simulink library "CSWLibrary"  (R2021a)
settings: Solver=VariableStepAuto  StartTime=0.0  StopTime=10.0  RelTol=1e-3
settings Model: Creator=Martin  LastModifiedBy=Martin

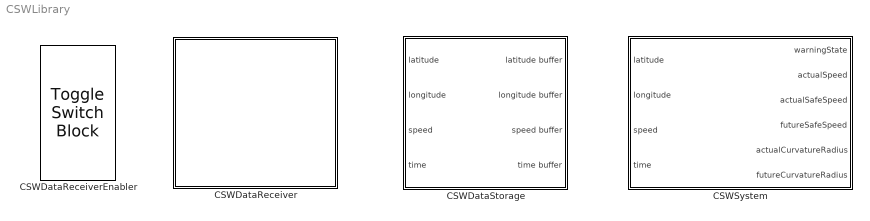
== system CSWLibrary ==
  CSWDataReceiver : MATLAB Function  TreatAsAtomicUnit=on  mask{inputPort=1, predictionTime=5, maximumLateralAcceleration=5.9, safeLimit=60, lowerRadius=20, upperRadius=600, isRunning=0, visualizeTrajectory=on, logReceivedData=on, receivedDataFile=output.xlsx, saveResults=on, simulationResultsFile=results.xlsx}
      mask prompts: inputPort "Serial port - COM"; predictionTime "Prediction time (s)"; maximumLateralAcceleration "Maximum lateral acceleration (m/s^2)"; safeLimit "Safe limit (0 -100%) of original Maximum lateral acceleration value"; lowerRadius "Lower limit (m)"; upperRadius "Upper limit (m)"; isRunning "Running"; visualizeTrajectory "Visualize trajectory - Future trajectory can be viewed by enabling checkbox."; logReceivedData "Log received data"; receivedDataFile "Received data file name (.xlsx)"; saveResults "Save simulation results"; simulationResultsFile "Results file name (.xlsx)"
      mask help:
      | CSWData receiver block of Curve Speed Warning System Toolbox processes received (online) GPS NMEA-0183 data from serial COM port. Data is used to simulate Curve Speed Warning system with options to visualize simulation, save received data and save simulation result data. Based on the input data, the system decides whether or not to give warning signal to driver. System is successfully initialized after getting 3 records containing correct input data.
      |
      | CSWData receiver block stops after CSWDataReceiver enabler block is set to Off value.
      |
      | CSWData receiver block expects online data.
  CSWDataReceiverEnabler : ToggleSwitchBlock
      settings: Values={{'Off', 'On'}, [0 1]}
  CSWDataStorage : Subsystem
      mask help:
      | CSWData storage block of Curve Speed Warning System Toolbox serves as storage for (offline) input data (latitude: double, longitude: double, speed: double, time: double) loaded from file, which are given as input data for CSWSystem block. Maximum capacity for each component of input data are 3 records.
      |
      | CSWData storage block is used to store offline data loaded from file.
  CSWSystem : MATLAB Function  TreatAsAtomicUnit=on  mask{predictionTime=5, maximumLateralAcceleration=5.9, safeLimit=60, lowerRadius=20, upperRadius=600, visualizeTrajectory=on, saveResults=on, simulationResultsFile=results.xlsx}
      mask prompts: predictionTime "Prediction time (s)"; maximumLateralAcceleration "Maximum lateral acceleration (m/s^2)"; safeLimit "Safe limit (0 -100%) of original Maximum lateral acceleration value"; lowerRadius "Lower limit (m)"; upperRadius "Upper limit (m)"; visualizeTrajectory "Visualize trajectory - Future trajectory can be viewed by enabling checkbox."; saveResults "Save simulation results"; simulationResultsFile "Results file name (.xlsx)"
      mask help:
      | System block of Curve Speed Warning System Toolbox processed input (offline) data (latitude: double, longitude: double, speed: double, time: double) from CSWData storage block to simulate Curve Speed Warning system. Data is used to simulate Curve Speed Warning system with options to visualize simulation and save simulation result data. Based on the input data, the system decides whether or not to give warning signal to driver. System is successfully initialized after getting 3 records containing correct input data.
      |
      | CSWSystem block expects offline data loaded from From Spreadsheet block with parameter Output after last data point set to Ground value.

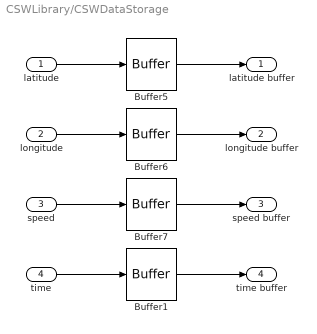
== system CSWLibrary/CSWDataStorage ==
  latitude : Inport
  longitude : Inport  Port=2
  speed : Inport  Port=3
  time : Inport  Port=4
  Buffer{1,5..7} (4 alike) : Buffer  N=3  V=2  ic=-199  OutputFrames=off
  latitude buffer : Outport
  longitude buffer : Outport  Port=2
  speed buffer : Outport  Port=3
  time buffer : Outport  Port=4
  wires:
  speed/1 -> Buffer7/1
  Buffer5/1 -> latitude buffer/1
  longitude/1 -> Buffer6/1
  Buffer7/1 -> speed buffer/1
  Buffer6/1 -> longitude buffer/1
  latitude/1 -> Buffer5/1
  time/1 -> Buffer1/1
  Buffer1/1 -> time buffer/1

== matlab function CSWLibrary/CSWSystem ==
  data: latitude input; longitude input; warningState output; actualSpeed output; actualSafeSpeed output; speed input; futureSafeSpeed output; actualCurvatureRadius output; futureCurvatureRadius output; time input
%% main function which represents Curve Speed Warning System uses loaded GPS data from file to compute simulation results which containts warning state, recommended speed etc.

function [warningState, actualSpeed, actualSafeSpeed, futureSafeSpeed, actualCurvatureRadius, futureCurvatureRadius] = CSWSystem(latitude,longitude,speed,time)
    coder.extrinsic('plot','legend','serialport','readline','nmeaParser','getfield','set_param','ceil','str2double',...
        'get_param','gcb','datetime');
    
    persistent predictionTime;  
    predictionTime = double(0);
    predictionTime = ceil(str2double(get_param(gcb,'predictionTime')));
    persistent maximumLateralAcceleration;
    maximumLateralAcceleration = double(0);
    maximumLateralAcceleration = str2double(get_param(gcb,'maximumLateralAcceleration'));
    persistent safeLimit;
    safeLimit = double(0);
    safeLimit = str2double(get_param(gcb,'safeLimit'));
    persistent lowerRadius;
    lowerRadius = double(0);
    lowerRadius = str2double(get_param(gcb,'lowerRadius'));
    persistent upperRadius;
    upperRadius = double(0);
    upperRadius = str2double(get_param(gcb,'upperRadius'));
    persistent visualizeTrajectory;
    visualizeTrajectory = str2bool(get_param(gcb,'visualizeTrajectory'));
    persistent saveResults;
    saveResults = str2bool(get_param(gcb,'saveResults'));
    
    % check if input data are valid
    validation(predictionTime, maximumLateralAcceleration, safeLimit, lowerRadius, upperRadius);
    
    % check if simulation results will be written to file
    persistent simulationResultsFile;  
    if(saveResults)
        simulationResultsFile = get_param(gcb,'simulationResultsFile');
        if(~endsWith(simulationResultsFile,'.xlsx'))
            error('Invalid simulation results file name format. Use .xlsx instead')
        end
    else
        simulationResultsFile = '-1';
    end

    persistent index;
    index = 3;
    
    data = [latitude(:) longitude(:) speed(:) time(:)];
    deltaTime12 = double(0);
    deltaTime23 = double(0);
    
    if ismember(-199, data)
        warningState = 0;
        actualSafeSpeed = -1;
        futureSafeSpeed = -1;
        actualCurvatureRadius = -1;
        futureCurvatureRadius = -1;
        actualSpeed = -1;
        return;
    end

    if (ismember(0, latitude(:)) && ismember(0, longitude(:)) && ismember(0, speed(:)) && ismember(0, time(:)))
        error('Input data contains an invalid zero value/s')
    end

    % convert coordinates to Cartesian coordinate system and center coordinates along Y axis
    data = centerDataArray(data);

    allData = [data(index - 2,1) data(index - 2,2) data(index - 2,3); 
        data(index - 1,1) data(index - 1,2) data(index - 1,3); 
        data(index,1) data(index,2) data(index,3)
        ];
    predictedData = [data(index,1) data(index,2) data(index,3)];

    tempData = [
        data(length(data(:,1))-2,1) data(length(data(:,1))-2,2) data(length(data(:,1))-2,3) data(length(data(:,1))-2,4);
        data(length(data(:,1))-1,1) data(length(data(:,1))-1,2) data(length(data(:,1))-1,3) data(length(data(:,1))-1,4); 
        data(length(data(:,1)),1) data(length(data(:,1)),2) data(length(data(:,1)),3) data(length(data(:,1)),4)
        ];
    
    % decode time values
    time1 = datetime(time(1),'ConvertFrom','posixtime', 'Format', 'yyyy-MM-dd HH:mm:ss');
    time2 = datetime(time(2),'ConvertFrom','posixtime', 'Format', 'yyyy-MM-dd HH:mm:ss');
    time3 = datetime(time(3),'ConvertFrom','posixtime', 'Format', 'yyyy-MM-dd HH:mm:ss');

    % differences between recording times
    deltaTime12 = seconds(diff(datetime([time1;time2])));
    deltaTime23 = seconds(diff(datetime([time2;time3])));
    
    % check validation of time differences (it's expected, that records will be received with same time frequency)
    if (deltaTime12 ~= deltaTime23)
        if(visualizeTrajectory)
            plot(0,0);
            title('invalid records, retrying...');
            set(gca, 'Color',[1 1 0]);
        end
        warningState = 0;
        actualSafeSpeed = -1;
        futureSafeSpeed = -1;
        actualCurvatureRadius = -1;
        futureCurvatureRadius = -1;
        actualSpeed = -1;
        return;
    end
    
    timeRate = deltaTime23;

    if (timeRate > 0)
        steps = 0;
        steps = ceil(predictionTime / timeRate);
        % prediction loop in which are future coordinates predicted
        for time = 1:steps
            [predictedX, predictedY] = predictCoordinates(tempData, 3, timeRate);  

            tempData = [tempData(2,1) tempData(2,2) tempData(2,3) tempData(2,4);
                tempData(3,1) tempData(3,2) tempData(3,3) tempData(3,4);
                predictedX predictedY getNextSpeed(tempData, 3) 0;
                ];

            allData = [allData; [tempData(3,1) tempData(3,2) tempData(3,3)]];
            predictedData = [predictedData; [tempData(3,1) tempData(3,2) tempData(3,3)]];
        end

        % compute radius and speed of actual and predicted data
        allData = computeCurvatureRadiusAndSpeed(allData,maximumLateralAcceleration*((100-safeLimit)/100));

        N = size(allData,1);
        allData = [allData,zeros(N,1)];

        % decide if warning should be invoked
        allData = checkCurvatureRadiusAndSpeed(allData, lowerRadius, upperRadius);
        
        % write results to file
        if(~isequal(simulationResultsFile,'-1'))
            writeResults(simulationResultsFile, allData, data(3,4));
        end

        actualSpeed = allData(3,3);
        actualSafeSpeed = allData(3,6);
        futureSafeSpeed = allData(4,6);
        actualCurvatureRadius = allData(3,5);
        futureCurvatureRadius = allData(4,5);

        if ismember(1, allData(:,7))
            warningState = 1;
        else
            warningState = 0;
        end
        
        % trajectory visualization containing referenced and predicted data
        if(visualizeTrajectory)
            plotOutput(allData, predictedData, timeRate);
        end
    else
        warningState = 0;
        actualSafeSpeed = -1;
        futureSafeSpeed = -1;
        actualCurvatureRadius = -1;
        futureCurvatureRadius = -1;
        actualSpeed = -1;
        return;
    end
end


%% convert string to boolean

function [output]=str2bool(string)
   if strcmp(string,'off')
     output = false;
   else
     output = true;
   end
end


%% input values validation

function validation(predictionTime, maximumLateralAcceleration, safeLimit, lowerRadius, upperRadius)
    if(predictionTime <= 0 || predictionTime > 30)
        error('Invalid value of prediction time. Valid value is from range 0(excluding) - 30')
    end
    
    if(maximumLateralAcceleration < 0)
        error('Negative value of maximum lateral acceleration is not supported')
    end
    
    if(safeLimit > 100 || safeLimit < 0)
        error('Invalid value of safe limit, set value in range 0 to 100')
    end
    
    if(lowerRadius < 0 || upperRadius < 0)
        error('Negative value of curvature radius limit is not supported')
    end

    if(lowerRadius > upperRadius)
        error('Lower limit of curvature radius must be smaller than upper limit')
    end
end


%% plot output prediction trajectory with / without warning

function plotOutput(allData, predictedData, timeRate)
    coder.extrinsic('plot','legend');
    
    % find maximum value among X,Y data points to specify size of plot figure
    xMin = min(allData(:,1)) - 5;
    xMax = max(allData(:,1)) + 5;
    
    x1 = abs(xMin);
    x2 = abs(xMax);
    
    xResult = x1;
    if(x1 < x2)
        xResult = x2;
    end
    
    yMin = min(allData(:,2)) - 5;
    yMax = max(allData(:,2)) + 5;
    
    y1 =  abs(yMin);
    y2 =  abs(yMax);
    
    yResult = y1;
    if(y1 < y2)
        yResult = y2;
    end
    
    result = 5;
    tempResult = yResult;
    if (yResult < xResult)
        tempResult = xResult;
    end
    if (result < tempResult)
        result = tempResult;
    end
    
    % plot output
    plot(allData(:,1), allData(:,2), 'b-o', 'DisplayName','referenced coordinates')
    xlim([-result result])
    ylim([yMin result])
    hold on
    plot(predictedData(:,1), predictedData(:,2), 'g-o', 'DisplayName','predicted coordinates')
    plot(predictedData(1,1), predictedData(1,2), 'k-o', 'DisplayName','actual position')
    
    % set frequency in which are points plotted in figure
    title(sprintf('point frequency is %.1f second/s',timeRate));
    
    % show figure legend
    legend('referenced coordinates','predicted coordinates','actual position')
    
    % set background color depending on warning state (warning - red background / no warning - white background)
    if ismember(1, allData(:,7))
        set(gca, 'Color',[1 0 0])
    else
        set(gca, 'Color',[1 1 1])
    end

    hold off
end


%% compute radius of curvature and recommended speed

function [predictedData] = computeCurvatureRadiusAndSpeed(predictedData,safeLimitOfLateralAcceleration)
    AlateralMax = safeLimitOfLateralAcceleration;

    [pathdistance,R,~] = curvature([predictedData(:,1) predictedData(:,2)]);
    predictedData = [predictedData pathdistance R];
    predictedData = [predictedData sqrt(predictedData(:, 5) * AlateralMax)];
end


%% Function circumcenter finds the radius R and the center of the circumscribed circle of a triangle in 3D space.  
%% reference to: https://uk.mathworks.com/matlabcentral/fileexchange/69452-curvature-of-a-1d-curve-in-a-2d-or-3d-space 

function [R,M,k] = circumcenter(A,B,C)
% Center and radius of the circumscribed circle for the triangle ABC
%  A,B,C  3D coordinate vectors for the triangle corners
%  R      Radius
%  M      3D coordinate vector for the center
%  k      Vector of length 1/R in the direction from A towards M
%         (Curvature vector)
  D = cross(B-A,C-A);
  b = norm(A-C);
  c = norm(A-B);
  if nargout == 1
    a = norm(B-C);     % slightly faster if only R is required
    R = a*b*c/2/norm(D);
    if norm(D) == 0
      R = Inf;
    end
    return
  end
  E = cross(D,B-A);
  F = cross(D,C-A); 
  G = (b^2*E-c^2*F)/norm(D)^2/2;
  M = A + G;
  R = norm(G);  % Radius of curvature
  if R == 0
    k = G;
  elseif norm(D) == 0
    R = Inf;
    k = D;
  else
    k = G'/R^2;   % Curvature vector
  end
end


%% Function curvature calls circumcenter for every triplet of neighboring points along the curve
%% reference to: https://uk.mathworks.com/matlabcentral/fileexchange/69452-curvature-of-a-1d-curve-in-a-2d-or-3d-space 

function [L,R,k] = curvature(input)
% Radius of curvature and curvature vector for 2D or 3D curve
%  [L,R,k] = curvature(X)
%   X:   2 or 3 column array of x, y (and possibly z) coordiates
%   L:   Cumulative arc length
%   R:   Radius of curvature
%   k:   Curvature vector
% The scalar curvature value is 1./R
% Version 2.6: Calculates end point values for closed curve
%   fefefe = X

  coder.varsize('X');
  coder.varsize('L');
  coder.varsize('R');
  coder.varsize('k');
  X = input;

  N = size(X,1);
  dims = size(X,2);
  if dims == 2
    X = [X,zeros(N,1)];  % Use 3D expressions for 2D as well
  end
  L = zeros(N,1);
  R = NaN(N,1);
  k = NaN(N,3);
  for i = 2:N-1
    [R(i),~,k(i,:)] = circumcenter(X(i,:)',X(i-1,:)',X(i+1,:)');
    L(i) = L(i-1)+norm(X(i,:)-X(i-1,:));
  end
  if norm(X(1,:)-X(end,:)) < 1e-10 % Closed curve. 
    [R(1),~,k(1,:)] = circumcenter(X(end-1,:)',X(1,:)',X(2,:)');
    R(end) = R(1);
    k(end,:) = k(1,:);
    L(end) = L(end-1) + norm(X(end,:)-X(end-1,:));
  end
  i = N;
  L(i) = L(i-1)+norm(X(i,:)-X(i-1,:));
  if dims == 2
    k = k(:,1:2);
  end
end


%% check if radius of curvature is valid and actual speed is higher than recommended

function [predictedData] = checkCurvatureRadiusAndSpeed(predictedData,lowerRadius,upperRadius)
    Rmin = lowerRadius;
    Rmax = upperRadius;
    
    for k=1:size(predictedData,1)
        
        % radius of curvature is invalid, not in range of <Rmin, Rmax>
        if predictedData(k,5) < Rmin || predictedData(k,5) > Rmax
            predictedData(k,7) = 0;
        else
            
            % actual speed is higher than recommended
            if predictedData(k,3) > predictedData(k,6)
                predictedData(k,7) = 1;
                
            % actual speed is lower than recommended
            else
                predictedData(k,7) = 0;
            end
        end
    end
end


%% compute angle between coordinates

function nextAngle = computeCoordinateAngle(data, index)
    % computes angle of referenced coordinates
    prevAngle = atan2( (data(index - 1,2) - data(index - 2,2)) , (data(index - 1,1) - data(index - 2,1)));
    actAngle = atan2( (data(index,2) - data(index - 1,2)) , (data(index,1) - data(index - 1,1)));
    
    % computes angle for predicted coordinates based on angle of referenced coordinates
    nextAngle = actAngle + (actAngle - prevAngle);
end


%% convert latitude, longitude to cartesian coordinate system

function [data] = convertDataArray(data)
    coder.extrinsic('latlon2local');
 
    % converts point locations given by lat, lon from geographic coordinates to local Cartesian coordinate system
    [xCoordinate, yCoordinate] = latlon2local(data(:,1), data(:,2), 0, [data(3,1), data(3,2), 0]);
    data = [xCoordinate yCoordinate data(:,3) data(:,4)];
end


%% center the coordinates along the y axis

function [data] = centerDataArray(data)
    centeredPoint = [0 1];
    
    data = convertDataArray(data);

    angle = atan2(centeredPoint(1,2) - data(3,2), centeredPoint(1,1) - data(3,1)) - atan2(data(2,2) - data(3,2), data(2,1) - data(3,1));
    result = deg2rad(180) - angle;

    x2 = data(2,1) * cos(result) + data(2,2) * sin(result);
    y2 = data(2,1) * -sin(result) + data(2,2) *  cos(result);

    x1 = data(1,1) * cos(result) + data(1,2) * sin(result);
    y1 = data(1,1) * -sin(result) + data(1,2) *  cos(result);

    centeredData = [x1 y1; x2 y2; data(3,1) data(3,2)];
    data(:,1) = centeredData(:,1);
    data(:,2) = centeredData(:,2);
end


%% get speed of actual position for predicted points

function [nextspeed] = getNextSpeed(data, index)
    nextspeed = data(index,3);
    if nextspeed < 0
        nextspeed = 0;
    end
end


%% predict coordinates

function [predictedX,predictedY] = predictCoordinates(data, index, time)
    speed = getNextSpeed(data, index);
    nextAngle = computeCoordinateAngle(data, index);

    predictedX = predictCoordinateX(data, index, nextAngle, time, speed);
    predictedY = predictCoordinateY(data, index, nextAngle, time, speed);
end


%% predict X coordinate

function predictedX = predictCoordinateX(data, index, angle, time, speed)
    predictedX = data(index,1) + speed * time * cos(angle);
end


%% predict Y coordinate

function predictedY = predictCoordinateY(data, index, angle, time, speed)
    predictedY = data(index,2) + speed * time * sin(angle);
end


%% write simulation results to file, Inf values are replaced by -1

function writeResults(simulationResultsFile, allData, tempTime)
    persistent resultsFileInitialized;
    coder.extrinsic('datetime','posixtime','table','writetable');
    time = datetime(tempTime,'ConvertFrom','posixtime', 'Format', 'yyyy-MM-dd HH:mm:ss');

    actualSpeed = allData(3,3);
    isInf = isinf(actualSpeed);
    actualSpeed(isInf) = -1;

    actualSafeSpeed = allData(3,6);
    isInf = isinf(actualSafeSpeed);
    actualSafeSpeed(isInf) = -1;

    futureSafeSpeed = allData(4,6);
    isInf = isinf(futureSafeSpeed);
    futureSafeSpeed(isInf) = -1;

    actualCurvatureRadius = allData(3,5);
    isInf = isinf(actualCurvatureRadius);
    actualCurvatureRadius(isInf) = -1;

    futureCurvatureRadius = allData(4,5);
    isInf = isinf(futureCurvatureRadius);
    futureCurvatureRadius(isInf) = -1;

    if ismember(1, allData(:,7))
        warningState = 1;
    else
        warningState = 0;
    end

    if isempty(resultsFileInitialized)
        writetable(table(time,warningState,actualSpeed,actualSafeSpeed,futureSafeSpeed,actualCurvatureRadius,futureCurvatureRadius,'VariableNames',{'time','warning','actual_speed','actual_recommended_speed','future_recommended_speed','actual_curvature_radius','future_curvature_radius'}),simulationResultsFile,"WriteMode",'overwritesheet',"AutoFitWidth",false);
        resultsFileInitialized = 1;
    else
        writetable(table(time,warningState,actualSpeed,actualSafeSpeed,futureSafeSpeed,actualCurvatureRadius,futureCurvatureRadius,'VariableNames',{'time','warning','actual_speed','actual_recommended_speed','future_recommended_speed','actual_curvature_radius','future_curvature_radius'}),simulationResultsFile,"WriteMode","append","AutoFitWidth",false);
    end
end

== matlab function CSWLibrary/CSWDataReceiver ==
%% main function which represents Curve Speed Warning System uses received GPS data from COM port to compute simulation results which containts warning state, recommended speed etc.

function CSWDataReceiver %#codegen
    coder.extrinsic('datestr', 'configureTerminator', 'serialport', 'read', 'readline', 'nmeaParser','getfield','set_param',...
        'strings','strrep','datenum','posixtime','str2double','get_param','gcb','append','plot','legend','ceil','gcb','datetime',...
        'writetable', 'table', 'endsWith');
    coder.varsize('data');
    
    persistent inputPort;
    inputPort = get_param(gcb,'inputPort');
    persistent predictionTime;  
    predictionTime = double(0);
    predictionTime = ceil(str2double(get_param(gcb,'predictionTime')));
    persistent maximumLateralAcceleration;
    maximumLateralAcceleration = double(0);
    maximumLateralAcceleration = str2double(get_param(gcb,'maximumLateralAcceleration'));
    persistent safeLimit;
    safeLimit = double(0);
    safeLimit = str2double(get_param(gcb,'safeLimit'));
    persistent lowerRadius;
    lowerRadius = double(0);
    lowerRadius = str2double(get_param(gcb,'lowerRadius'));
    persistent upperRadius;
    upperRadius = double(0);
    upperRadius = str2double(get_param(gcb,'upperRadius'));
    persistent visualizeTrajectory;
    visualizeTrajectory = str2bool(get_param(gcb,'visualizeTrajectory'));
    persistent logReceivedData;
    logReceivedData = str2bool(get_param(gcb,'logReceivedData'));
    persistent saveResults;
    saveResults = str2bool(get_param(gcb,'saveResults'));
    
    % check if input data are valid
    validation(predictionTime, maximumLateralAcceleration, safeLimit, lowerRadius, upperRadius);
     
    % check if received data / simulation results will be written to file
    persistent receivedDataFile;   
    if(logReceivedData)
        receivedDataFile = get_param(gcb,'receivedDataFile');
        if(~endsWith(receivedDataFile,'.xlsx'))
            error('Invalid received data file name format. Use .xlsx instead')
        end
    else
        receivedDataFile = '-1';
    end
    
    persistent simulationResultsFile;  
    if(saveResults)
        simulationResultsFile = get_param(gcb,'simulationResultsFile');
        if(~endsWith(simulationResultsFile,'.xlsx'))
            error('Invalid simulation results file name format. Use .xlsx instead')
        end
    else
        simulationResultsFile = '-1';
    end

    % receiver and NMEA parser initialization
    PORT = append("COM",inputPort);
    device = serialport(PORT,4800,'Timeout',3);
    pnmea = nmeaParser("MessageIDs", "RMC");
    
    isRunning = get_param(gcb,'isRunning');
    
    persistent flag;
    flag = 1;
    persistent index;
    index = 3;
    data = [];
    originalData = [];
    deltaTime12 = double(0);
    deltaTime23 = double(0);
    
    %% Main program loop
    while isequal(isRunning,'1') 
        % read received data
        record = readline(device);
        isRunning = get_param(gcb,'isRunning');
        
        % received data validation
        if ~isempty(record)

            % fill data structure with initialization data
            if isempty(data) || (~isempty(data) && length(data(:,1)) ~= index)
                data = updateDataArray(receivedDataFile, data, record, pnmea, 1);
            else
                if flag
                    originalData = data;
                    flag = 0;
                end
                originalData = updateDataArray(receivedDataFile, originalData, record, pnmea, 0);
                data = originalData;
                
                % convert coordinates to Cartesian coordinate system and center coordinates along Y axis
                data = centerDataArray(data);

                allData = [data(index - 2,1) data(index - 2,2) data(index - 2,3); 
                    data(index - 1,1) data(index - 1,2) data(index - 1,3); 
                    data(index,1) data(index,2) data(index,3)
                    ];
                predictedData = [data(index,1) data(index,2) data(index,3)];

                tempData = [
                    data(length(data(:,1))-2,1) data(length(data(:,1))-2,2) data(length(data(:,1))-2,3) data(length(data(:,1))-2,4);
                    data(length(data(:,1))-1,1) data(length(data(:,1))-1,2) data(length(data(:,1))-1,3) data(length(data(:,1))-1,4); 
                    data(length(data(:,1)),1) data(length(data(:,1)),2) data(length(data(:,1)),3) data(length(data(:,1)),4)
                    ];

                % decode time values
                time1 = datetime(data(1,4),'ConvertFrom','posixtime', 'Format', 'yyyy-MM-dd HH:mm:ss');
                time2 = datetime(data(2,4),'ConvertFrom','posixtime', 'Format', 'yyyy-MM-dd HH:mm:ss');
                time3 = datetime(data(3,4),'ConvertFrom','posixtime', 'Format', 'yyyy-MM-dd HH:mm:ss');

                % differences between recording times
                deltaTime12 = seconds(diff(datetime([time1;time2])));
                deltaTime23 = seconds(diff(datetime([time2;time3])));

                % check validation of time differences (it's expected, that records will be received with same time frequency)
                if (deltaTime12 ~= deltaTime23)
                    if(visualizeTrajectory)
                        plot(0,0);
                        title('invalid records, retrying...');
                        set(gca, 'Color',[1 1 0]);
                    end
                else
                    timeRate = deltaTime23;

                    if (timeRate > 0)
                        steps = 0;
                        steps = ceil(predictionTime / timeRate);

                        % prediction loop in which are future coordinates predicted
                        for time = 1:steps
                            [predictedX, predictedY] = predictCoordinates(tempData, 3, timeRate);  

                            tempData = [tempData(2,1) tempData(2,2) tempData(2,3) tempData(2,4);
                                tempData(3,1) tempData(3,2) tempData(3,3) tempData(3,4);
                                predictedX predictedY getNextSpeed(tempData, 3) 0;
                                ];

                            allData = [allData; [tempData(3,1) tempData(3,2) tempData(3,3)]];
                            predictedData = [predictedData; [tempData(3,1) tempData(3,2) tempData(3,3)]];
                        end

                        % compute radius and speed of actual and predicted data
                        allData = computeCurvatureRadiusAndSpeed(allData,maximumLateralAcceleration*((100-safeLimit)/100));

                        N = size(allData,1);
                        allData = [allData,zeros(N,1)];

                        % decide if warning should be invoked
                        allData = checkCurvatureRadiusAndSpeed(allData, lowerRadius, upperRadius);

                        % write results to file
                        if(~isequal(simulationResultsFile,'-1'))
                            writeResults(simulationResultsFile, allData, data(3,4));
                        end

                        % trajectory visualization containing referenced and predicted data
                        if(visualizeTrajectory)
                            plotOutput(allData, predictedData, timeRate);
                        end
                    else
                        continue
                    end
                end
            end
        end
        record = readline(device);
    end
end


%% convert string to boolean

function output = str2bool(string)
   if strcmp(string,'off')
     output = false;
   else
     output = true;
   end
end


%% input values validation

function validation(predictionTime, maximumLateralAcceleration, safeLimit, lowerRadius, upperRadius)
    if(predictionTime <= 0 || predictionTime > 30)
        error('Invalid value of prediction time. Valid value is from range 0(excluding) - 30')
    end
    
    if(maximumLateralAcceleration < 0)
        error('Negative value of maximum lateral acceleration is not supported')
    end
    
    if(safeLimit > 100 || safeLimit < 0)
        error('Invalid value of safe limit, set value in range 0 to 100')
    end
    
    if(lowerRadius < 0 || upperRadius < 0)
        error('Negative value of curvature radius limit is not supported')
    end

    if(lowerRadius > upperRadius)
        error('Lower limit of curvature radius must be smaller than upper limit')
    end
end


%% plot output prediction trajectory with / without warning

function plotOutput(allData, predictedData, timeRate)
    coder.extrinsic('plot','legend');
    
    % find maximum value among X,Y data points to specify size of plot figure
    xMin = min(allData(:,1)) - 5;
    xMax = max(allData(:,1)) + 5;
    
    x1 = abs(xMin);
    x2 = abs(xMax);
    
    xResult = x1;
    if(x1 < x2)
        xResult = x2;
    end
    
    yMin = min(allData(:,2)) - 5;
    yMax = max(allData(:,2)) + 5;
    
    y1 =  abs(yMin);
    y2 =  abs(yMax);
    
    yResult = y1;
    if(y1 < y2)
        yResult = y2;
    end
    
    result = 5;
    tempResult = yResult;
    if (yResult < xResult)
        tempResult = xResult;
    end
    if (result < tempResult)
        result = tempResult;
    end
    
    % plot output
    plot(allData(:,1), allData(:,2), 'b-o', 'DisplayName','referenced coordinates')
    xlim([-result result])
    ylim([yMin result])
    hold on
    plot(predictedData(:,1), predictedData(:,2), 'g-o', 'DisplayName','predicted coordinates')
    plot(predictedData(1,1), predictedData(1,2), 'k-o', 'DisplayName','actual position')
    
    % set frequency in which are points plotted in figure
    title(sprintf('point frequency is %.1f second/s',timeRate));
    
    % show figure legend
    legend('referenced coordinates','predicted coordinates','actual position')
    
    % set background color depending on warning state (warning - red background / no warning - white background)
    if ismember(1, allData(:,7))
        set(gca, 'Color',[1 0 0])
    else
        set(gca, 'Color',[1 1 1])
    end

    hold off
end


%% compute radius of curvature and recommended speed

function predictedData = computeCurvatureRadiusAndSpeed(predictedData,safeLimitOfLateralAcceleration)
    AlateralMax = safeLimitOfLateralAcceleration;

    [pathdistance,R,~] = curvature([predictedData(:,1) predictedData(:,2)]);
    predictedData = [predictedData pathdistance R];
    predictedData = [predictedData sqrt(predictedData(:, 5) * AlateralMax)];
end


%% Function circumcenter finds the radius R and the center of the circumscribed circle of a triangle in 3D space.  
%% reference to: https://uk.mathworks.com/matlabcentral/fileexchange/69452-curvature-of-a-1d-curve-in-a-2d-or-3d-space 

function [R,M,k] = circumcenter(A,B,C)
% Center and radius of the circumscribed circle for the triangle ABC
%  A,B,C  3D coordinate vectors for the triangle corners
%  R      Radius
%  M      3D coordinate vector for the center
%  k      Vector of length 1/R in the direction from A towards M
%         (Curvature vector)
  D = cross(B-A,C-A);
  b = norm(A-C);
  c = norm(A-B);
  if nargout == 1
    a = norm(B-C);     % slightly faster if only R is required
    R = a*b*c/2/norm(D);
    if norm(D) == 0
      R = Inf;
    end
    return
  end
  E = cross(D,B-A);
  F = cross(D,C-A); 
  G = (b^2*E-c^2*F)/norm(D)^2/2;
  M = A + G;
  R = norm(G);  % Radius of curvature
  if R == 0
    k = G;
  elseif norm(D) == 0
    R = Inf;
    k = D;
  else
    k = G'/R^2;   % Curvature vector
  end
end


%% Function curvature calls circumcenter for every triplet of neighboring points along the curve
%% reference to: https://uk.mathworks.com/matlabcentral/fileexchange/69452-curvature-of-a-1d-curve-in-a-2d-or-3d-space 

function [L,R,k] = curvature(input)
% Radius of curvature and curvature vector for 2D or 3D curve
%  [L,R,k] = curvature(X)
%   X:   2 or 3 column array of x, y (and possibly z) coordiates
%   L:   Cumulative arc length
%   R:   Radius of curvature
%   k:   Curvature vector
% The scalar curvature value is 1./R
% Version 2.6: Calculates end point values for closed curve
%   fefefe = X

  coder.varsize('X');
  coder.varsize('L');
  coder.varsize('R');
  coder.varsize('k');
  X = input;

  N = size(X,1);
  dims = size(X,2);
  if dims == 2
    X = [X,zeros(N,1)];  % Use 3D expressions for 2D as well
  end
  L = zeros(N,1);
  R = NaN(N,1);
  k = NaN(N,3);
  for i = 2:N-1
    [R(i),~,k(i,:)] = circumcenter(X(i,:)',X(i-1,:)',X(i+1,:)');
    L(i) = L(i-1)+norm(X(i,:)-X(i-1,:));
  end
  if norm(X(1,:)-X(end,:)) < 1e-10 % Closed curve. 
    [R(1),~,k(1,:)] = circumcenter(X(end-1,:)',X(1,:)',X(2,:)');
    R(end) = R(1);
    k(end,:) = k(1,:);
    L(end) = L(end-1) + norm(X(end,:)-X(end-1,:));
  end
  i = N;
  L(i) = L(i-1)+norm(X(i,:)-X(i-1,:));
  if dims == 2
    k = k(:,1:2);
  end
end


%% check if radius of curvature is valid and actual speed is higher than recommended

function predictedData = checkCurvatureRadiusAndSpeed(predictedData,lowerRadius,upperRadius)
    Rmin = lowerRadius;
    Rmax = upperRadius;
    
    for k=1:size(predictedData,1)
        
        % radius of curvature is invalid, not in range of <Rmin, Rmax>
        if predictedData(k,5) < Rmin || predictedData(k,5) > Rmax
            predictedData(k,7) = 0;
        else
            
            % actual speed is higher than recommended
            if predictedData(k,3) > predictedData(k,6)
                predictedData(k,7) = 1;
                
            % actual speed is lower than recommended
            else
                predictedData(k,7) = 0;
            end
        end
    end
end


%% compute angle between coordinates

function nextAngle = computeCoordinateAngle(data, index)
    % compute angle of referenced coordinates
    prevAngle = atan2( (data(index - 1,2) - data(index - 2,2)) , (data(index - 1,1) - data(index - 2,1)));
    actAngle = atan2( (data(index,2) - data(index - 1,2)) , (data(index,1) - data(index - 1,1)));
    
    % compute angle for predicted coordinates based on angle of referenced coordinates
    nextAngle = actAngle + (actAngle - prevAngle);
end


%% convert latitude, longitude to cartesian coordinate system

function data = convertDataArray(data)
    coder.extrinsic('latlon2local');
 
    % convert point locations given by lat, lon from geographic coordinates to local Cartesian coordinate system
    [xCoordinate, yCoordinate] = latlon2local(data(:,1), data(:,2), 0, [data(3,1), data(3,2), 0]);
    data = [xCoordinate yCoordinate data(:,3) data(:,4)];
end


%% center the coordinates along the y axis

function data = centerDataArray(data)
    centeredPoint = [0 1];
    
    data = convertDataArray(data);

    angle = atan2(centeredPoint(1,2) - data(3,2), centeredPoint(1,1) - data(3,1)) - atan2(data(2,2) - data(3,2), data(2,1) - data(3,1));
    result = deg2rad(180) - angle;

    x2 = data(2,1) * cos(result) + data(2,2) * sin(result);
    y2 = data(2,1) * -sin(result) + data(2,2) *  cos(result);

    x1 = data(1,1) * cos(result) + data(1,2) * sin(result);
    y1 = data(1,1) * -sin(result) + data(1,2) *  cos(result);

    centeredData = [x1 y1; x2 y2; data(3,1) data(3,2)];
    data(:,1) = centeredData(:,1);
    data(:,2) = centeredData(:,2);
end


%% get speed of actual position for predicted points

function nextspeed = getNextSpeed(data, index)
    nextspeed = data(index,3);
    if nextspeed < 0
        nextspeed = 0;
    end
end


%% predict coordinates

function [predictedX,predictedY] = predictCoordinates(data, index, time)
    speed = getNextSpeed(data, index);
    nextAngle = computeCoordinateAngle(data, index);

    predictedX = predictCoordinateX(data, index, nextAngle, time, speed);
    predictedY = predictCoordinateY(data, index, nextAngle, time, speed);
end


%% predict X coordinate

function predictedX = predictCoordinateX(data, index, angle, time, speed)
    predictedX = data(index,1) + speed * time * cos(angle);
end


%% predict Y coordinate

function predictedY = predictCoordinateY(data, index, angle, time, speed)
    predictedY = data(index,2) + speed * time * sin(angle);
end


%% insert / update data structure by GPS data

function data = updateDataArray(fileName, data, record, pnmea, insertData)
    persistent outputFileInitialized;
    coder.extrinsic('getfield','isequal','posixtime','table','writetable');
    
    % convert NMEA-0183 record
    nmeaRecord = pnmea(record);
    
    % preinitialize variables
    latitude=zeros(1,1);
    longitude=zeros(1,1);
    speed=zeros(1,1);
    time=zeros(1,1);
    status=zeros(1,1);
    
    % parse NMEA-0183 record
    latitude = getfield(nmeaRecord,'Latitude');
    longitude = getfield(nmeaRecord,'Longitude');
    speed = getfield(nmeaRecord,'GroundSpeed');
    tempTime = getfield(nmeaRecord,'UTCDateTime');
    status = double(getfield(nmeaRecord,'Status'));

    % input data validation
    if isequal(status,0) && ~isnan(latitude) && ~isnan(longitude) && ~isnan(speed)
        % save data to output file
        if(~isequal(fileName,'-1'))
            if isempty(outputFileInitialized)
                writetable(table(latitude,longitude,speed,tempTime,'VariableNames',{'latitude','longitude','speed','time'}),fileName,"WriteMode",'overwritesheet',"AutoFitWidth",false);
                outputFileInitialized = 1;
            else
                writetable(table(latitude,longitude,speed,tempTime,'VariableNames',{'latitude','longitude','speed','time'}),fileName,"WriteMode","append","AutoFitWidth",false);
            end
        end
        
        % insert GPS data to data structure
        if isequal(insertData,1)
            time = posixtime(tempTime);
            data = [data; latitude longitude speed time];
            
        % update data structure
        else
            time = posixtime(tempTime);

            tempData = [data(2,1) data(2,2) data(2,3) data(2,4); 
                data(3,1) data(3,2) data(3,3) data(3,4); 
                latitude longitude speed time];
            data = tempData;
        end
    end
end


%% write simulation results to file, Inf values are replaced by -1

function writeResults(simulationResultsFile, allData, tempTime)
    persistent resultsFileInitialized;
    coder.extrinsic('datetime','posixtime','table','writetable');
    time = datetime(tempTime,'ConvertFrom','posixtime', 'Format', 'yyyy-MM-dd HH:mm:ss');

    actualSpeed = allData(3,3);
    isInf = isinf(actualSpeed);
    actualSpeed(isInf) = -1;

    actualSafeSpeed = allData(3,6);
    isInf = isinf(actualSafeSpeed);
    actualSafeSpeed(isInf) = -1;

    futureSafeSpeed = allData(4,6);
    isInf = isinf(futureSafeSpeed);
    futureSafeSpeed(isInf) = -1; 

    actualCurvatureRadius = allData(3,5);
    isInf = isinf(actualCurvatureRadius);
    actualCurvatureRadius(isInf) = -1;

    futureCurvatureRadius = allData(4,5);
    isInf = isinf(futureCurvatureRadius);
    futureCurvatureRadius(isInf) = -1;

    if ismember(1, allData(:,7))
        warningState = 1;
    else
        warningState = 0;
    end

    if isempty(resultsFileInitialized)
        writetable(table(time,warningState,actualSpeed,actualSafeSpeed,futureSafeSpeed,actualCurvatureRadius,futureCurvatureRadius,'VariableNames',{'time','warning','actual_speed','actual_recommended_speed','future_recommended_speed','actual_curvature_radius','future_curvature_radius'}),simulationResultsFile,"WriteMode",'overwritesheet',"AutoFitWidth",false);
        resultsFileInitialized = 1;
    else
        writetable(table(time,warningState,actualSpeed,actualSafeSpeed,futureSafeSpeed,actualCurvatureRadius,futureCurvatureRadius,'VariableNames',{'time','warning','actual_speed','actual_recommended_speed','future_recommended_speed','actual_curvature_radius','future_curvature_radius'}),simulationResultsFile,"WriteMode","append","AutoFitWidth",false);
    end
end
